simulink model "modelul2"  (R2022b)
settings: Solver=VariableStepAuto  StartTime=0.0  StopTime=30  RelTol=1e-3
undefined symbols (not defined in the file or in its folder): par
settings Model: Creator=zuch3e  LastModifiedBy=zuch3e
settings DataIOCC: ReturnWorkspaceOutputs=off

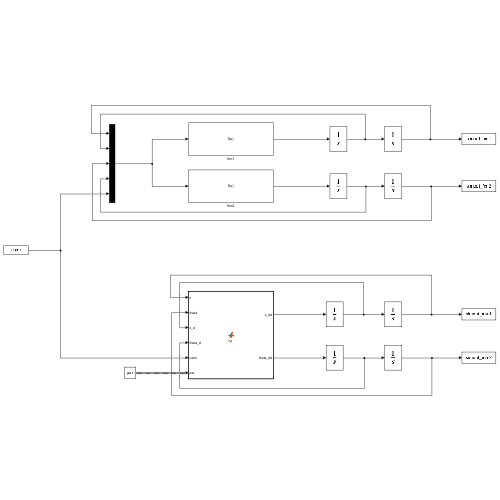
[thumbnail: Simulink's stored preview of the top-level diagram]
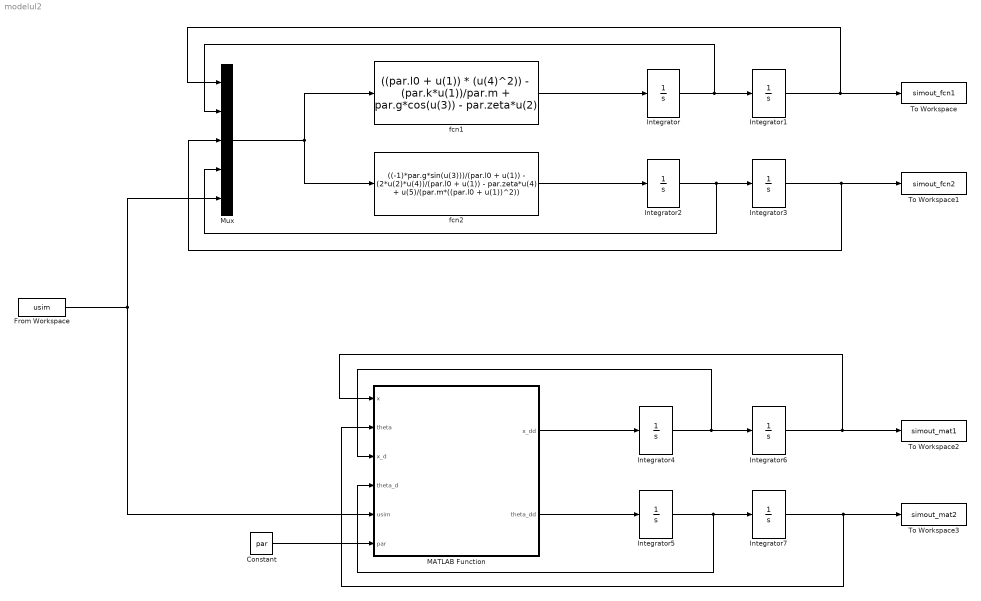
== system modelul2 ==
  Constant : Constant  Value=par  OutDataTypeStr=Bus: par_bus
  From Workspace : FromWorkspace  VariableName=usim
  Integrator{,1..7} (8 alike) : Integrator
  MATLAB Function : MATLAB Function  TreatAsAtomicUnit=on
  Mux : Mux  Inputs=5
  To Workspace : ToWorkspace  VariableName=simout_fcn1  SaveFormat=Timeseries  SampleTime=-1
  To Workspace1 : ToWorkspace  VariableName=simout_fcn2  SaveFormat=Timeseries  SampleTime=-1
  To Workspace2 : ToWorkspace  VariableName=simout_mat1  SaveFormat=Timeseries  SampleTime=-1
  To Workspace3 : ToWorkspace  VariableName=simout_mat2  SaveFormat=Timeseries  SampleTime=-1
  fcn1 : Fcn  Expr=((par.l0 + u(1)) * (u(4)^2)) - (par.k*u(1))/par.m + par.g*cos(u(3)) - par.zeta*u(2)
  fcn2 : Fcn  Expr=((-1)*par.g*sin(u(3)))/(par.l0 + u(1)) - (2*u(2)*u(4))/(par.l0 + u(1)) - par.zeta*u(4) + u(5)/(par.m*((par.l0 + u(1))^2))
  wires:
  fcn1/1 -> Integrator/1
  Integrator/1 -> Mux/2, Integrator1/1
  Integrator1/1 -> Mux/1, To Workspace/1
  fcn2/1 -> Integrator2/1
  Integrator2/1 -> Mux/4, Integrator3/1
  Integrator3/1 -> Mux/3, To Workspace1/1
  Mux/1 -> fcn2/1, fcn1/1
  From Workspace/1 -> MATLAB Function/5(usim), Mux/5
  MATLAB Function/1(x_dd) -> Integrator4/1
  Integrator4/1 -> MATLAB Function/3(x_d), Integrator6/1
  Integrator6/1 -> MATLAB Function/1(x), To Workspace2/1
  Integrator7/1 -> MATLAB Function/2(theta), To Workspace3/1
  Integrator5/1 -> MATLAB Function/4(theta_d), Integrator7/1
  MATLAB Function/2(theta_dd) -> Integrator5/1
  Constant/1 -> MATLAB Function/6(par)

== matlab function modelul2/MATLAB Function ==
  data: x input; x_dd output; theta input; x_d input; theta_d input; usim input; par input; theta_dd output
function [x_dd, theta_dd] = fcn(x,theta,x_d,theta_d,usim, par)
x_dd = ((par.l0 + x) * (theta_d^2)) - (par.k*x)/par.m + par.g*cos(theta) - par.zeta*x_d;
theta_dd = ((-1)*par.g*sin(theta))/(par.l0 + x) - (2*x_d*theta_d)/(par.l0 + x) - par.zeta*theta_d + usim/(par.m*((par.l0 + x)^2));
end
